simulink model "simulink_controller"  (R2024b)
settings: Solver=FixedStepAuto  StartTime=0.0  StopTime=30  RelTol=1e-3
values from neighbouring files (symbols this model uses):
  A = [1 0 T -0.5*T^2 0 ... (first row only)    [mpc_data.m]
  B = [0; 0; 0; T/tau; 1/tau]    [mpc_data.m]
  C = [1 -th 0 0  0 ... (first row only)    [mpc_data.m]
  T = 0.2    [mpc_data.m]
settings Model: Creator=Aylar  LastModifiedBy=Aylar

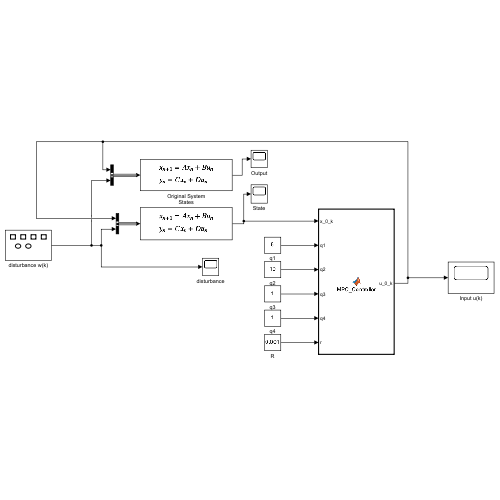
[thumbnail: Simulink's stored preview of the top-level diagram]
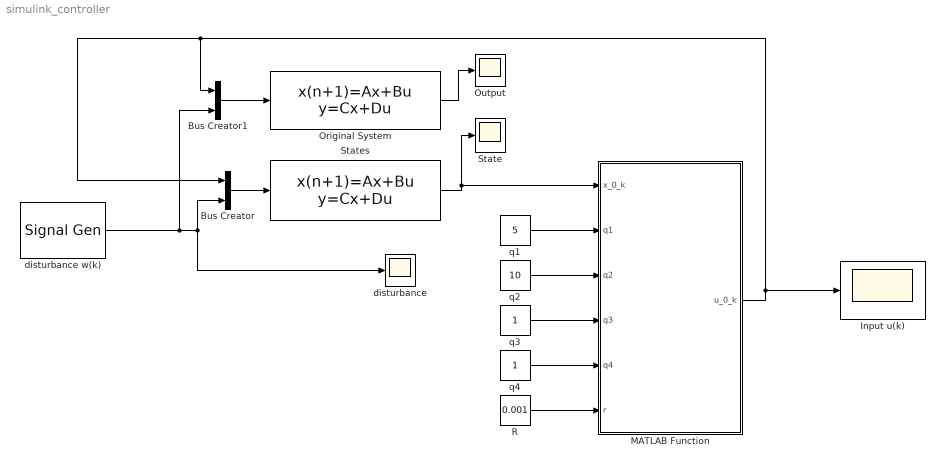
== system simulink_controller ==
  Bus Creator : BusCreator  Inputs=2
  Bus Creator1 : BusCreator  Inputs=2
  Input u(k) : Scope
  MATLAB Function : MATLAB Function  TreatAsAtomicUnit=on
  Original System : DiscreteStateSpace  A=A  B=[B,E]  C=C  D=zeros(4,2)  InitialCondition=[100;30;-10;0;0]  SampleTime=T
  Output : Scope
  R : Constant  Value=0.001
  State : Scope
  States : DiscreteStateSpace  A=A  B=[B,E]  C=eye(5)  D=zeros(5,2)  InitialCondition=[100;30;-10;0;0]  SampleTime=T
  disturbance : Scope
  disturbance w(k) : SignalGenerator  WaveForm=square  Amplitude=0  Frequency=0.1  Units=rad/sec
  q1 : Constant  Value=5
  q2 : Constant  Value=10
  q3 : Constant
  q4 : Constant
  wires:
  States/1 -> MATLAB Function/1(x_0_k), State/1
  Original System/1 -> Output/1
  q1/1 -> MATLAB Function/2(q1)
  q2/1 -> MATLAB Function/3(q2)
  q3/1 -> MATLAB Function/4(q3)
  q4/1 -> MATLAB Function/5(q4)
  R/1 -> MATLAB Function/6(r)
  Bus Creator/1 -> States/1
  Bus Creator1/1 -> Original System/1
  MATLAB Function/1(u_0_k) -> Input u(k)/1, Bus Creator1/1, Bus Creator/1
  disturbance w(k)/1 -> Bus Creator1/2, Bus Creator/2, disturbance/1

== matlab function simulink_controller/MATLAB Function ==
  data: x_0_k input; u_0_k output; q1 input; q2 input; q3 input; q4 input; r input
function u_0_k = MPC_Controller(x_0_k, q1, q2, q3, q4, r)
%#codegen
persistent G H C1 Qbar Rbar F1 F2 F3 F4 F5 Cbar S2 S4 S5 V1 V2_p V3_p V4_p V5_p d0

if isempty(G)
s = coder.load('mpc_data.mat', 'G','H', 'C1', 'Qbar','Rbar',...
    'F1','F2','F3','F4','F5','Cbar','S2','S4','S5',...
    'V1','V2_p','V3_p','V4_p','V5_p', 'd0');

G = s.G; H = s.H; C1 = s.C1; Qbar = s.Qbar; Rbar = s.Rbar;
F1 = s.F1; F2 = s.F2; F3 = s.F3; F4 = s.F4; F5 = s.F5;
Cbar = s.Cbar; S2 = s.S2; S4 = s.S4; S5 = s.S5;
V1 = s.V1; V2_p = s.V2_p; V3_p = s.V3_p; V4_p = s.V4_p; V5_p = s.V5_p; d0 = s.d0;

end

F = [F1; F2; F3; F4; F5];

V2 = V2_p - -C1*H*x_0_k;
V3 = V3_p - [S2; -S2]*H*x_0_k;
V4 = V4_p - [S4; -S4]*H*x_0_k;
V5 = V5_p - [S5; -S5]*H*x_0_k;
    
V = [V1; V2; V3; V4; V5];

M = (Cbar*G)'*Qbar*(Cbar*G)+Rbar;
H_qp = M;

f_qp = 2* (Cbar*H*x_0_k-repmat([d0; 0;0;0], 11, 1))'*Qbar * Cbar* G;
A_qp = F;
b_qp = V;



% Empty matrices for unused inputs
Aeq = [];
beq = [];
lb = [];
ub = [];

% Options: use active-set algorithm (required)
options = optimoptions('quadprog', 'Algorithm', 'active-set', 'Display', 'off');

% Initial guess
n = size(H_qp, 1);
x0 = zeros(n,1);

% Full 10-argument call
u_seq = quadprog(H_qp, f_qp, A_qp, b_qp, Aeq, beq, lb, ub, x0, options);


u_0_k = u_seq(1);

end
